simulink model "InverseKinematics_TESTMODELL"  (R2024a)
settings: Solver=VariableStepAuto  StartTime=0.0  StopTime=10.0  RelTol=1e-3
undefined symbols (not defined in the file or in its folder): l1, l2
settings Model: Creator=apaul  LastModifiedBy=apaul

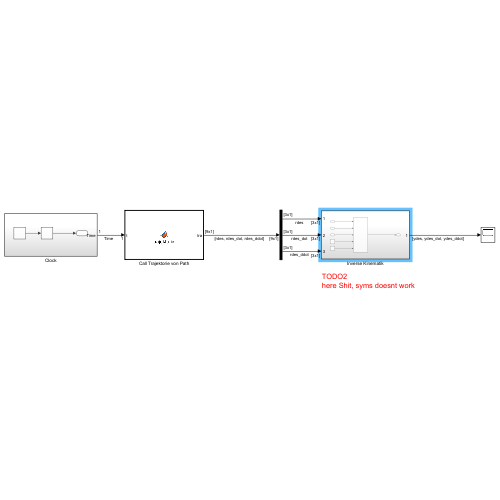
[thumbnail: Simulink's stored preview of the top-level diagram]
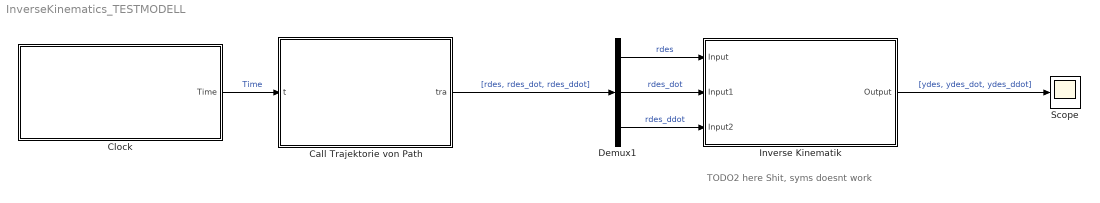
== system InverseKinematics_TESTMODELL ==
  note: TODO2
      | here Shit, syms doesnt work
  Call Trajektorie von Path : MATLAB Function  TreatAsAtomicUnit=on
  Clock : Subsystem
  Demux1 : Demux  Outputs=3
  Inverse Kinematik : Subsystem
  Scope : Scope
  wires:
  Demux1/2 -> Inverse Kinematik/2(Input1)  "rdes_dot"
  Clock/1(Time) -> Call Trajektorie von Path/1(t)  "Time"
  Demux1/3 -> Inverse Kinematik/3(Input2)  "rdes_ddot"
  Demux1/1 -> Inverse Kinematik/1(Input)  "rdes"
  Call Trajektorie von Path/1(tra) -> Demux1/1  "[rdes, rdes_dot, rdes_ddot]"
  Inverse Kinematik/1(Output) -> Scope/1  "[ydes, ydes_dot, ydes_ddot]"

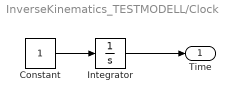
== system InverseKinematics_TESTMODELL/Clock ==
  Constant : Constant
  Integrator : Integrator
  Time : Outport
  wires:
  Constant/1 -> Integrator/1
  Integrator/1 -> Time/1

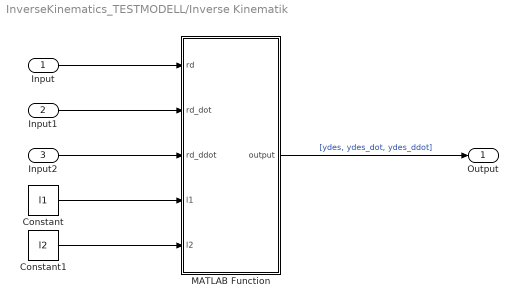
== system InverseKinematics_TESTMODELL/Inverse Kinematik ==
  Input : Inport
  Input1 : Inport  Port=2
  Input2 : Inport  Port=3
  Constant : Constant  Value=l1
  Constant1 : Constant  Value=l2
  MATLAB Function : MATLAB Function  TreatAsAtomicUnit=on
  Output : Outport
  wires:
  Input/1 -> MATLAB Function/1(rd)
  MATLAB Function/1(output) -> Output/1  "[ydes, ydes_dot, ydes_ddot]"
  Input1/1 -> MATLAB Function/2(rd_dot)
  Input2/1 -> MATLAB Function/3(rd_ddot)
  Constant/1 -> MATLAB Function/4(l1)
  Constant1/1 -> MATLAB Function/5(l2)

== matlab function InverseKinematics_TESTMODELL/Inverse Kinematik/MATLAB Function ==
  data: rd input; output output; rd_dot input; rd_ddot input; l1 input; l2 input
function output = fcn(rd,rd_dot,rd_ddot,l1,l2)
%SHIT, I don t want to do integration, but technically i could define
%alpha0 beta0 and shit and then compute the numerical shit then integrate
%and ... but annoying

%LSG via optimazation
%could feed in y...

%just say al,beta = 0 for initial guess
T_0EF = T_0EF_fcn(alpha,beta,l1,l2);

r = T_0EF(1:3,4);

error = norm(rd - r);

% Optimization options
options = optimoptions('fminunc', 'Display', 'iter', 'Algorithm', 'quasi-newton');

%initial guess
y0 = [0;0];

[alpha, beta] = fminunc(@(theta) objectiveFunction(theta, target, L), y0, options);

J = Jfunc()

    
yd = [alpha; beta];
yd_dot = [0;0];
yd_ddot = [0;0];
output = [yd; yd_dot; yd_ddot];
end

== matlab function InverseKinematics_TESTMODELL/Call Trajektorie von Path ==
  data: tra output; t input
function tra = trajektorie(t)
%Trajektorie
tra = CALCtrajektorie(t);
end
